simulink model "task_13_simulink"  (R2021b)
settings: Solver=VariableStepAuto  StartTime=0.0  StopTime=10.0  RelTol=1e-3
settings Model: Creator=aleksejshevcenko  LastModifiedBy=aleksejshevcenko

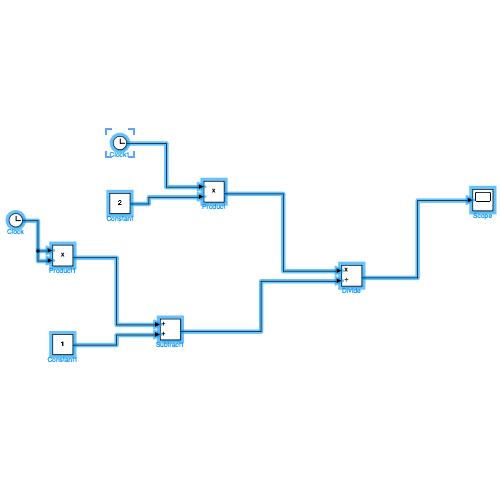
[thumbnail: Simulink's stored preview of the top-level diagram]
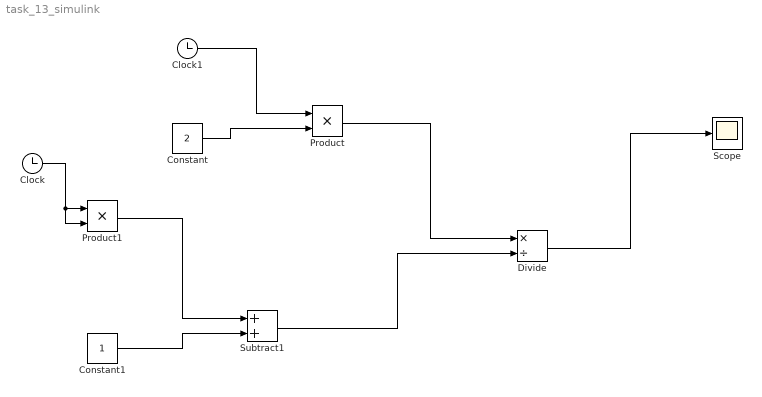
== system task_13_simulink ==
  Clock : Clock
  Clock1 : Clock
  Constant : Constant  Value=2
  Constant1 : Constant
  Divide : Product  Inputs=*/
  Product : Product
  Product1 : Product
  Scope : Scope
  Subtract1 : Sum
  wires:
  Divide/1 -> Scope/1
  Constant/1 -> Product/2
  Clock1/1 -> Product/1
  Constant1/1 -> Subtract1/2
  Product1/1 -> Subtract1/1
  Clock/1 -> Product1/1, Product1/2
  Subtract1/1 -> Divide/2
  Product/1 -> Divide/1
